simulink library "tpm"  (R2021b)
settings: Solver=VariableStepAuto  StartTime=0.0  StopTime=10.0  RelTol=1e-3
undefined symbols (not defined in the file or in its folder): ENUM_AN_LF, ENUM_AN_LR, ENUM_AN_RF, ENUM_AN_RR, ENUM_POWERSTA_OFF, ENUM_POWERSTA_OFFA, ENUM_POWERSTA_OFFC, ENUM_POWERSTA_ON, ENUM_POWERSTA_READY, ENUM_POWERSTA_STANDBY, ENUM_PWRSTASW_OFF, ENUM_PWRSTASW_OFFA, ENUM_PWRSTASW_OFFCHVCHRG, ENUM_PWRSTASW_STANDBY, KTPM_Delay_raw8, KTPM_WhlRotDir_enum_ovrdflg, KTPM_WhlRotDir_enum_ovrdval, TRUE, ZERO_FLOAT, ZERO_INT
libraries: simulink x58, hcu_lib x25, $bdroot x18
(part 5 of 8)

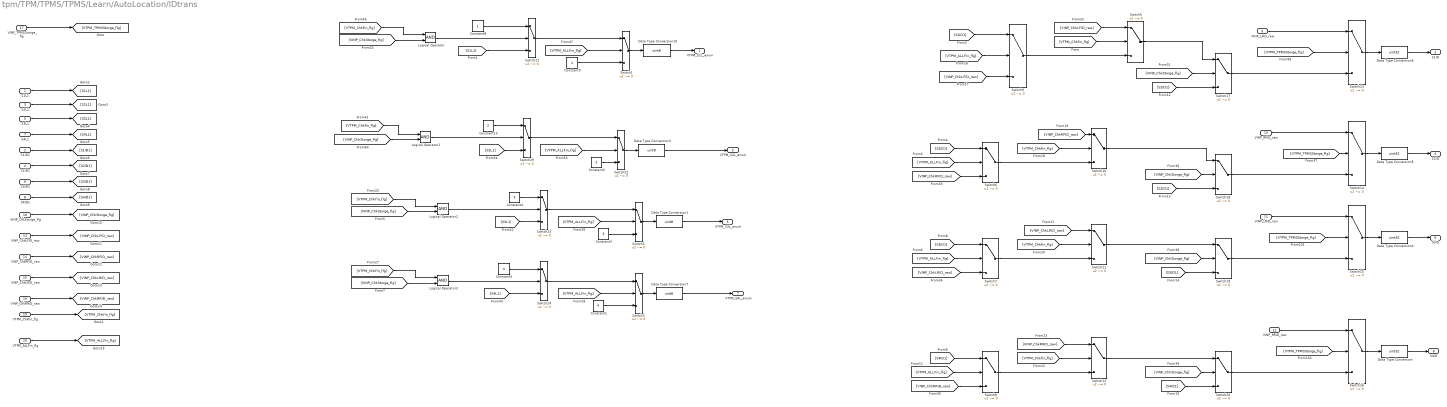
== system tpm/TPM/TPMS/TPMS/Learn/AutoLocation/IDtrans ==
  S1L1 : Inport
  S1ID1 : Inport  Port=2
  S2L1 : Inport  Port=3
  S2ID1 : Inport  Port=4
  S3L1 : Inport  Port=5
  S3ID1 : Inport  Port=6
  S4L1 : Inport  Port=7
  S4ID1 : Inport  Port=8
  VINP_LFID_raw : Inport  Port=9
  VINP_RFID_raw : Inport  Port=10
  VINP_LRID_raw : Inport  Port=11
  VINP_RRID_raw : Inport  Port=12
  VINP_ChkLFID_raw : Inport  Port=13
  VINP_ChkRFID_raw : Inport  Port=14
  VINP_ChkLRID_raw : Inport  Port=15
  VINP_ChkRRID_raw : Inport  Port=16
  VINP_TPMSStorge_flg : Inport  Port=17
  VINP_ChkStorge_flg : Inport  Port=18
  VTPM_Chkfin_flg : Inport  Port=19
  VTPM_ALLFin_flg : Inport  Port=20
  Constant1 : Constant  Value=4
  Constant13 : Constant  Value=2
  Constant2 : Constant  Value=2
  Constant3 : Constant  Value=3
  Constant4 : Constant  Value=3
  Constant5 : Constant  Value=4
  Constant8 : Constant
  Constant9 : Constant
  Data Type Conversion{,4..6} (4 alike) : DataTypeConversion  OutDataTypeStr=uint32
  Data Type Conversion{1,3,7,10} (4 alike) : DataTypeConversion  OutDataTypeStr=uint8
  Logical Operator{,1..3} (4 alike) : Logic  AllPortsSameDT=off  OutDataTypeStr=boolean
  Switch{1..3,5..24,29} (24 alike) : Switch  Criteria=u2 ~= 0
  VTPM_S1L_enum : Outport
  S1ID : Outport  Port=2
  VTPM_S2L_enum : Outport  Port=3
  S2ID : Outport  Port=4
  VTPM_S3L_enum : Outport  Port=5
  S3ID : Outport  Port=6
  VTPM_S4L_enum : Outport  Port=7
  S4ID : Outport  Port=8
  wires:
  Data Type Conversion4/1 -> S3ID/1
  Data Type Conversion6/1 -> S1ID/1
  Data Type Conversion/1 -> S4ID/1
  [VTPM_TPMSStorge_flg] -> Switch13/2
  Data Type Conversion5/1 -> S2ID/1
  VINP_TPMSStorge_flg/1 -> [VTPM_TPMSStorge_flg]
  S1L1/1 -> [S1L1]
  S2L1/1 -> [S2L1]
  S3L1/1 -> [S3L1]
  S4L1/1 -> [S4L1]
  S1ID1/1 -> [S1ID1]
  S2ID1/1 -> [S2ID1]
  S3ID1/1 -> [S3ID1]
  S4ID1/1 -> [S4ID1]
  VINP_LFID_raw/1 -> Switch13/1
  [VTPM_TPMSStorge_flg] -> Switch14/2
  Switch14/1 -> Data Type Conversion5/1
  Switch18/1 -> Switch14/3
  [VTPM_TPMSStorge_flg] -> Switch15/2
  VINP_LRID_raw/1 -> Switch15/1
  Switch19/1 -> Switch15/3
  Switch15/1 -> Data Type Conversion4/1
  VINP_RRID_raw/1 -> Switch16/1
  [VTPM_TPMSStorge_flg] -> Switch16/2
  Switch16/1 -> Data Type Conversion/1
  Switch13/1 -> Data Type Conversion6/1
  VINP_ChkStorge_flg/1 -> [VINP_ChkStorge_flg]
  VINP_ChkLFID_raw/1 -> [VINP_ChkLFID_raw]
  VINP_ChkRFID_raw/1 -> [VINP_ChkRFID_raw]
  VINP_ChkLRID_raw/1 -> [VINP_ChkLRID_raw]
  VINP_ChkRRID_raw/1 -> [VINP_ChkRRID_raw]
  [S1ID1] -> Switch17/3
  [VINP_ChkStorge_flg] -> Switch17/2
  [S2ID1] -> Switch18/3
  [VINP_ChkStorge_flg] -> Switch18/2
  [VINP_ChkStorge_flg] -> Switch19/2
  [S3ID1] -> Switch19/3
  [VINP_ChkStorge_flg] -> Switch20/2
  [S4ID1] -> Switch20/3
  Switch17/1 -> Switch13/3
  VINP_RFID_raw/1 -> Switch14/1
  Switch20/1 -> Switch16/3
  VTPM_ALLFin_flg/1 -> [VTPM_ALLFin_flg]
  VTPM_Chkfin_flg/1 -> [VTPM_Chkfin_flg]
  Switch5/1 -> Switch17/1
  [VTPM_Chkfin_flg] -> Switch5/2
  [VINP_ChkRFID_raw] -> Switch6/3
  [VTPM_ALLFin_flg] -> Switch6/2
  [S2ID1] -> Switch6/1
  [VINP_ChkLRID_raw] -> Switch7/3
  [VTPM_ALLFin_flg] -> Switch7/2
  [S3ID1] -> Switch7/1
  [S4ID1] -> Switch8/1
  [VINP_ChkRRID_raw] -> Switch8/3
  [VTPM_ALLFin_flg] -> Switch8/2
  [VTPM_ALLFin_flg] -> Switch9/2
  [S1ID1] -> Switch9/1
  [VINP_ChkLFID_raw] -> Switch9/3
  [VINP_ChkLFID_raw] -> Switch5/1
  Switch9/1 -> Switch5/3
  Switch10/1 -> Switch18/1
  [VTPM_Chkfin_flg] -> Switch10/2
  Switch6/1 -> Switch10/3
  [VINP_ChkRFID_raw] -> Switch10/1
  Switch11/1 -> Switch19/1
  Switch7/1 -> Switch11/3
  [VTPM_Chkfin_flg] -> Switch11/2
  [VINP_ChkLRID_raw] -> Switch11/1
  [VTPM_Chkfin_flg] -> Switch12/2
  Switch12/1 -> Switch20/1
  Switch8/1 -> Switch12/3
  [VINP_ChkRRID_raw] -> Switch12/1
  Switch1/1 -> Data Type Conversion10/1
  Data Type Conversion10/1 -> VTPM_S1L_enum/1
  [VTPM_ALLFin_flg] -> Switch1/2
  Switch21/1 -> Switch1/1
  Constant9/1 -> Switch1/3
  Constant8/1 -> Switch21/1
  Logical Operator/1 -> Switch21/2
  [VTPM_Chkfin_flg] -> Logical Operator/1
  [VINP_ChkStorge_flg] -> Logical Operator/2
  [S1L1] -> Switch21/3
  [VTPM_Chkfin_flg] -> Logical Operator1/1
  Switch29/1 -> Switch22/1
  Switch22/1 -> Data Type Conversion3/1
  Logical Operator1/1 -> Switch29/2
  [VTPM_ALLFin_flg] -> Switch22/2
  [VINP_ChkStorge_flg] -> Logical Operator1/2
  Data Type Conversion3/1 -> VTPM_S2L_enum/1
  Constant2/1 -> Switch22/3
  Constant13/1 -> Switch29/1
  [S2L1] -> Switch29/3
  [VTPM_Chkfin_flg] -> Logical Operator2/1
  Switch23/1 -> Switch2/1
  Switch2/1 -> Data Type Conversion1/1
  Logical Operator2/1 -> Switch23/2
  [VTPM_ALLFin_flg] -> Switch2/2
  [VINP_ChkStorge_flg] -> Logical Operator2/2
  Constant3/1 -> Switch2/3
  Data Type Conversion1/1 -> VTPM_S3L_enum/1
  Constant4/1 -> Switch23/1
  [S3L1] -> Switch23/3
  [VTPM_Chkfin_flg] -> Logical Operator3/1
  Switch24/1 -> Switch3/1
  Switch3/1 -> Data Type Conversion7/1
  Logical Operator3/1 -> Switch24/2
  [VTPM_ALLFin_flg] -> Switch3/2
  [VINP_ChkStorge_flg] -> Logical Operator3/2
  Data Type Conversion7/1 -> VTPM_S4L_enum/1
  Constant1/1 -> Switch3/3
  [S4L1] -> Switch24/3
  Constant5/1 -> Switch24/1

== system tpm/TPM/TPMS/TPMS/Learn/AutoLocation/Subsystem ==
  S1ID : Inport
  S2ID : Inport  Port=2
  S3ID : Inport  Port=3
  S4ID : Inport  Port=4
  VINP_TPMSResButt_flg : Inport  Port=5
  Enable : EnablePort
  Chart : Stateflow chart  TreatAsAtomicUnit=on
  VTPM_FlashS1ID_raw : Outport
  VTPM_FlashS2ID_raw : Outport  Port=2
  VTPM_FlashS3ID_raw : Outport  Port=3
  VTPM_FlashS4ID_raw : Outport  Port=4
  VTPM_FlashIDvalid_enum : Outport  Port=5
  wires:
  S4ID/1 -> Chart/4(S4ID)
  VINP_TPMSResButt_flg/1 -> Chart/5(VINP_TPMSResButt_flg)
  S3ID/1 -> Chart/3(S3ID)
  S2ID/1 -> Chart/2(S2ID)
  S1ID/1 -> Chart/1(S1ID)
  Chart/5(VTPM_FlashIDvalid_enum) -> VTPM_FlashIDvalid_enum/1
  Chart/4(VTPM_FlashS4ID_raw) -> VTPM_FlashS4ID_raw/1
  Chart/3(VTPM_FlashS3ID_raw) -> VTPM_FlashS3ID_raw/1
  Chart/2(VTPM_FlashS2ID_raw) -> VTPM_FlashS2ID_raw/1
  Chart/1(VTPM_FlashS1ID_raw) -> VTPM_FlashS1ID_raw/1

== system tpm/TPM/TPMS/TPMS/Learn/AutoLocation/WheelPosition ==
  VPMM_PowerSta_enum : Inport
  VINP_LFPulseCountV_flg : Inport  Port=2
  VTPM_LFWhlRotDir_enum : Inport  Port=3
  VINP_LFPulseCount_cnt : Inport  Port=4
  VINP_RFPulseCountV_flg : Inport  Port=5
  VTPM_RFWhlRotDir_enum : Inport  Port=6
  VINP_RFPulseCount_cnt : Inport  Port=7
  VINP_LRPulseCountV_flg : Inport  Port=8
  VTPM_LRWhlRotDir_enum : Inport  Port=9
  VINP_LRPulseCount_cnt : Inport  Port=10
  VINP_RRPulseCountV_flg : Inport  Port=11
  VTPM_RRWhlRotDir_enum : Inport  Port=12
  VINP_RRPulseCount_cnt : Inport  Port=13
  Chart1 : Stateflow chart
      settings: PortSchema="{\"entries\":[{\"content\":{\"sides\":[{\"content\":{\"connectorIds\":[\"In1\",\"In3\",\"In4\",\"In2\"]},\"type\":\"ConnectorPlacement.EquallySpacedRectSide\",\"uuid\":\"75b213f6-e1d2-4b51-b3b2-bb9425a07129\"},{\"content\":{\"connectorIds\":[\"Out1\"],\"side\":\"RIGHT\"},\"type\":\"ConnectorPlacement.EquallySpacedRectSide\",\"uuid\":\"38a0f576-9623-4928-9f9d-a0457630f06b\"},{\"content\":{\"connectorIds\":[],\"side\":\"TOP\"},\"type\":\"ConnectorPlacement.EquallySpacedRectSide\",\"uuid\":\"5f96c838-eaaa-41a3-a60b-23098d5837b3\"}]},\"type\":\"ConnectorPlacement.EquallySpacedConnector\",\"uuid\":\"5c398a97-3ae6-4872-b8e8-e03a196625be\"}],\"packageUris\":[\"http://schema.mathworks.com/mf0/Connector/R2020b\"],\"version\":\"1.0\"}"
  Chart2 : Stateflow chart
      settings: PortSchema="{\"entries\":[{\"content\":{\"sides\":[{\"content\":{\"connectorIds\":[\"In1\",\"In3\",\"In4\",\"In2\"]},\"type\":\"ConnectorPlacement.EquallySpacedRectSide\",\"uuid\":\"75b213f6-e1d2-4b51-b3b2-bb9425a07129\"},{\"content\":{\"connectorIds\":[\"Out1\"],\"side\":\"RIGHT\"},\"type\":\"ConnectorPlacement.EquallySpacedRectSide\",\"uuid\":\"38a0f576-9623-4928-9f9d-a0457630f06b\"},{\"content\":{\"connectorIds\":[],\"side\":\"TOP\"},\"type\":\"ConnectorPlacement.EquallySpacedRectSide\",\"uuid\":\"5f96c838-eaaa-41a3-a60b-23098d5837b3\"}]},\"type\":\"ConnectorPlacement.EquallySpacedConnector\",\"uuid\":\"5c398a97-3ae6-4872-b8e8-e03a196625be\"}],\"packageUris\":[\"http://schema.mathworks.com/mf0/Connector/R2020b\"],\"version\":\"1.0\"}"
  Chart3 : Stateflow chart
      settings: PortSchema="{\"entries\":[{\"content\":{\"sides\":[{\"content\":{\"connectorIds\":[\"In1\",\"In3\",\"In4\",\"In2\"]},\"type\":\"ConnectorPlacement.EquallySpacedRectSide\",\"uuid\":\"75b213f6-e1d2-4b51-b3b2-bb9425a07129\"},{\"content\":{\"connectorIds\":[\"Out1\"],\"side\":\"RIGHT\"},\"type\":\"ConnectorPlacement.EquallySpacedRectSide\",\"uuid\":\"38a0f576-9623-4928-9f9d-a0457630f06b\"},{\"content\":{\"connectorIds\":[],\"side\":\"TOP\"},\"type\":\"ConnectorPlacement.EquallySpacedRectSide\",\"uuid\":\"5f96c838-eaaa-41a3-a60b-23098d5837b3\"}]},\"type\":\"ConnectorPlacement.EquallySpacedConnector\",\"uuid\":\"5c398a97-3ae6-4872-b8e8-e03a196625be\"}],\"packageUris\":[\"http://schema.mathworks.com/mf0/Connector/R2020b\"],\"version\":\"1.0\"}"
  Chart5 : Stateflow chart
      settings: PortSchema="{\"entries\":[{\"content\":{\"sides\":[{\"content\":{\"connectorIds\":[\"In1\",\"In3\",\"In4\",\"In2\"]},\"type\":\"ConnectorPlacement.EquallySpacedRectSide\",\"uuid\":\"75b213f6-e1d2-4b51-b3b2-bb9425a07129\"},{\"content\":{\"connectorIds\":[\"Out1\"],\"side\":\"RIGHT\"},\"type\":\"ConnectorPlacement.EquallySpacedRectSide\",\"uuid\":\"38a0f576-9623-4928-9f9d-a0457630f06b\"},{\"content\":{\"connectorIds\":[],\"side\":\"TOP\"},\"type\":\"ConnectorPlacement.EquallySpacedRectSide\",\"uuid\":\"5f96c838-eaaa-41a3-a60b-23098d5837b3\"}]},\"type\":\"ConnectorPlacement.EquallySpacedConnector\",\"uuid\":\"5c398a97-3ae6-4872-b8e8-e03a196625be\"}],\"packageUris\":[\"http://schema.mathworks.com/mf0/Connector/R2020b\"],\"version\":\"1.0\"}"
  Subsystem : Subsystem
  Subsystem1 : Subsystem
  Subsystem2 : Subsystem
  Subsystem3 : Subsystem
  VTPM_RFWP_raw16 : Outport
  VTPM_LRWP_raw16 : Outport  Port=2
  VTPM_RRWP_raw16 : Outport  Port=3
  VTPM_LFWP_raw16 : Outport  Port=4
  wires:
  VPMM_PowerSta_enum/1 -> [VPMM_PowerSta_enum]
  [VPMM_PowerSta_enum] -> Chart1/1(VPMM_PowerSta_enum)
  [VPMM_PowerSta_enum] -> Chart2/1(VPMM_PowerSta_enum)
  [VPMM_PowerSta_enum] -> Chart3/1(VPMM_PowerSta_enum)
  VINP_LFPulseCountV_flg/1 -> Chart1/3(VINP_LFPulseCountV_flg)
  VTPM_LFWhlRotDir_enum/1 -> Chart1/4(VTPM_LFWhlRotDir_enum)
  VINP_LFPulseCount_cnt/1 -> Chart1/2(VINP_LFPulseCount_cnt)
  VINP_RFPulseCountV_flg/1 -> Chart2/3(VINP_RFPulseCountV_flg)
  VTPM_RFWhlRotDir_enum/1 -> Chart2/4(VTPM_RFWhlRotDir_enum)
  VINP_RFPulseCount_cnt/1 -> Chart2/2(VINP_RFPulseCount_cnt)
  VINP_LRPulseCountV_flg/1 -> Chart3/3(VINP_LRPulseCountV_flg)
  VTPM_LRWhlRotDir_enum/1 -> Chart3/4(VTPM_LRWhlRotDir_enum)
  VINP_LRPulseCount_cnt/1 -> Chart3/2(VINP_LRPulseCount_cnt)
  Subsystem/1(VTPM_LFWP_raw16) -> VTPM_LFWP_raw16/1
  Subsystem1/1(VTPM_RFWP_raw16) -> VTPM_RFWP_raw16/1
  Subsystem2/1(VTPM_LRWP_raw16) -> VTPM_LRWP_raw16/1
  Subsystem3/1(VTPM_RRWP_raw16) -> VTPM_RRWP_raw16/1
  Chart1/1(VTPM_LFWpos_raw) -> Subsystem/1(VTPM_LFWpos_raw)  "VTPM_LFWpos_raw"
  Chart2/1(VTPM_RFWpos_raw) -> Subsystem1/1(VTPM_RFWpos_raw)  "VTPM_RFWpos_raw"
  Chart3/1(VTPM_LRWpos_raw) -> Subsystem2/1(VTPM_LRWpos_raw)  "VTPM_LRWpos_raw"
  [VPMM_PowerSta_enum] -> Chart5/1(VPMM_PowerSta_enum)
  VINP_RRPulseCountV_flg/1 -> Chart5/3(VINP_RRPulseCountV_flg)
  VTPM_RRWhlRotDir_enum/1 -> Chart5/4(VTPM_RRWhlRotDir_enum)
  VINP_RRPulseCount_cnt/1 -> Chart5/2(VINP_RRPulseCount_cnt)
  Chart5/1(VTPM_RRWpos_raw) -> Subsystem3/1(VTPM_RRWpos_raw)  "VTPM_RRWpos_raw"

== system tpm/TPM/TPMS/TPMS/Send/Alarm/LFTHighWarn ==
  VTPM_LFWheelTemp_C : Inport
  Compare To Constant : simulink/Logic and Bit Operations/Compare To Constant  relop=>=  const=90  OutDataTypeStr=boolean
  Compare To Constant1 : simulink/Logic and Bit Operations/Compare To Constant  relop=>=  const=84  OutDataTypeStr=boolean
  Logical Operator1 : Logic  Operator=OR  AllPortsSameDT=off  OutDataTypeStr=boolean
  Logical Operator2 : Logic  AllPortsSameDT=off  OutDataTypeStr=boolean
  Unit Delay : UnitDelay  SampleTime=-1  HasFrameUpgradeWarning=on
  VTPM_LFWheelTmpIndi_flg : Outport
  wires:
  Compare To Constant/1 -> Logical Operator1/1
  Unit Delay/1 -> Logical Operator2/2
  Logical Operator2/1 -> Logical Operator1/2
  Logical Operator1/1 -> VTPM_LFWheelTmpIndi_flg/1, Unit Delay/1
  Compare To Constant1/1 -> Logical Operator2/1
  VTPM_LFWheelTemp_C/1 -> Compare To Constant/1, Compare To Constant1/1

== system tpm/TPM/TPMS/TPMS/Send/Alarm/LRTHighWarn ==
  VTPM_LRWheelTemp_C : Inport
  Compare To Constant : simulink/Logic and Bit Operations/Compare To Constant  relop=>=  const=90  OutDataTypeStr=boolean
  Compare To Constant1 : simulink/Logic and Bit Operations/Compare To Constant  relop=>=  const=84  OutDataTypeStr=boolean
  Logical Operator1 : Logic  Operator=OR  AllPortsSameDT=off  OutDataTypeStr=boolean
  Logical Operator2 : Logic  AllPortsSameDT=off  OutDataTypeStr=boolean
  Unit Delay : UnitDelay  SampleTime=-1  HasFrameUpgradeWarning=on
  VTPM_LRWheelTmpIndi_flg : Outport
  wires:
  Compare To Constant/1 -> Logical Operator1/1
  Unit Delay/1 -> Logical Operator2/2
  Logical Operator2/1 -> Logical Operator1/2
  Logical Operator1/1 -> VTPM_LRWheelTmpIndi_flg/1, Unit Delay/1
  Compare To Constant1/1 -> Logical Operator2/1
  VTPM_LRWheelTemp_C/1 -> Compare To Constant/1, Compare To Constant1/1

== system tpm/TPM/TPMS/TPMS/Send/Alarm/RFTHighWarn ==
  VTPM_RFWheelTemp_C : Inport
  Compare To Constant : simulink/Logic and Bit Operations/Compare To Constant  relop=>=  const=90  OutDataTypeStr=boolean
  Compare To Constant1 : simulink/Logic and Bit Operations/Compare To Constant  relop=>=  const=84  OutDataTypeStr=boolean
  Logical Operator1 : Logic  Operator=OR  AllPortsSameDT=off  OutDataTypeStr=boolean
  Logical Operator2 : Logic  AllPortsSameDT=off  OutDataTypeStr=boolean
  Unit Delay : UnitDelay  SampleTime=-1  HasFrameUpgradeWarning=on
  VTPM_RFWheelTmpIndi_flg : Outport
  wires:
  VTPM_RFWheelTemp_C/1 -> Compare To Constant1/1, Compare To Constant/1
  Compare To Constant1/1 -> Logical Operator2/1
  Logical Operator1/1 -> VTPM_RFWheelTmpIndi_flg/1, Unit Delay/1
  Logical Operator2/1 -> Logical Operator1/2
  Unit Delay/1 -> Logical Operator2/2
  Compare To Constant/1 -> Logical Operator1/1

== system tpm/TPM/TPMS/TPMS/Send/Alarm/RRTHighWarn ==
  VTPM_RRWheelTemp_C : Inport
  Compare To Constant : simulink/Logic and Bit Operations/Compare To Constant  relop=>=  const=90  OutDataTypeStr=boolean
  Compare To Constant1 : simulink/Logic and Bit Operations/Compare To Constant  relop=>=  const=84  OutDataTypeStr=boolean
  Logical Operator1 : Logic  Operator=OR  AllPortsSameDT=off  OutDataTypeStr=boolean
  Logical Operator2 : Logic  AllPortsSameDT=off  OutDataTypeStr=boolean
  Unit Delay : UnitDelay  SampleTime=-1  HasFrameUpgradeWarning=on
  VTPM_RRWheelTmpIndi_flg : Outport
  wires:
  VTPM_RRWheelTemp_C/1 -> Compare To Constant1/1, Compare To Constant/1
  Compare To Constant1/1 -> Logical Operator2/1
  Logical Operator1/1 -> VTPM_RRWheelTmpIndi_flg/1, Unit Delay/1
  Logical Operator2/1 -> Logical Operator1/2
  Unit Delay/1 -> Logical Operator2/2
  Compare To Constant/1 -> Logical Operator1/1

== system tpm/TPM/TPMS/TPMS/Send/DATA/LocationSW ==
  VTPM_S1ID_raw32 : Inport
  VTPM_S2ID_raw32 : Inport  Port=2
  VTPM_S3ID_raw32 : Inport  Port=3
  VTPM_S4ID_raw32 : Inport  Port=4
  VINP_IDin_raw32 : Inport  Port=5
  VTPM_S1L_enum : Inport  Port=6
  VTPM_S2L_enum : Inport  Port=7
  VTPM_S3L_enum : Inport  Port=8
  VTPM_S4L_enum : Inport  Port=9
  VINP_DATAin_flg : Inport  Port=10
  VTPM_IDLOCK_flg : Inport  Port=11
  Chart1 : Stateflow chart  TreatAsAtomicUnit=on
  VTPM_LFSW_flg : Outport
  VTPM_RFSW_flg : Outport  Port=2
  VTPM_LRSW_flg : Outport  Port=3
  VTPM_RRSW_flg : Outport  Port=4
  wires:
  VTPM_S1ID_raw32/1 -> Chart1/1(VTPM_S1ID_raw32)
  VTPM_S1L_enum/1 -> Chart1/2(VTPM_S1L_enum)
  VTPM_S2ID_raw32/1 -> Chart1/3(VTPM_S2ID_raw32)
  VTPM_S2L_enum/1 -> Chart1/4(VTPM_S2L_enum)
  VTPM_S3ID_raw32/1 -> Chart1/5(VTPM_S3ID_raw32)
  VTPM_S3L_enum/1 -> Chart1/6(VTPM_S3L_enum)
  VTPM_S4ID_raw32/1 -> Chart1/7(VTPM_S4ID_raw32)
  VTPM_S4L_enum/1 -> Chart1/8(VTPM_S4L_enum)
  VINP_IDin_raw32/1 -> Chart1/9(VINP_IDin_raw32)
  VINP_DATAin_flg/1 -> Chart1/10(VINP_DATAin_flg)
  Chart1/1(VTPM_LFSW_flg) -> VTPM_LFSW_flg/1
  Chart1/2(VTPM_RFSW_flg) -> VTPM_RFSW_flg/1
  Chart1/3(VTPM_LRSW_flg) -> VTPM_LRSW_flg/1
  Chart1/4(VTPM_RRSW_flg) -> VTPM_RRSW_flg/1
  VTPM_IDLOCK_flg/1 -> Chart1/11(VTPM_IDLOCK_flg)

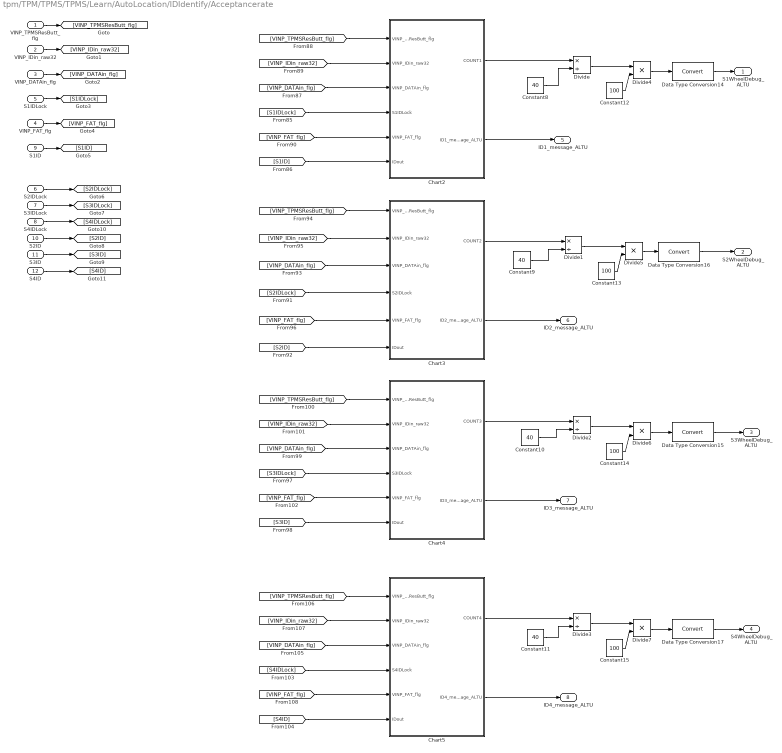
== system tpm/TPM/TPMS/TPMS/Learn/AutoLocation/IDIdentify/Acceptancerate ==
  VINP_TPMSResButt_flg : Inport
  VINP_IDin_raw32 : Inport  Port=2
  VINP_DATAin_flg : Inport  Port=3
  VINP_FAT_flg : Inport  Port=4
  S1IDLock : Inport  Port=5
  S2IDLock : Inport  Port=6
  S3IDLock : Inport  Port=7
  S4IDLock : Inport  Port=8
  S1ID : Inport  Port=9
  S2ID : Inport  Port=10
  S3ID : Inport  Port=11
  S4ID : Inport  Port=12
  Chart2 : Stateflow chart  TreatAsAtomicUnit=on
      settings: PortSchema="{\"entries\":[{\"content\":{\"sides\":[{\"content\":{\"connectorIds\":[\"In2\",\"In1\",\"In3\",\"In4\",\"In5\",\"In6\"]},\"type\":\"ConnectorPlacement.EquallySpacedRectSide\",\"uuid\":\"0106c0c7-b0dd-4985-8477-027279f2cfbe\"},{\"content\":{\"connectorIds\":[\"Out1\",\"Out2\"],\"side\":\"RIGHT\"},\"type\":\"ConnectorPlacement.EquallySpacedRectSide\",\"uuid\":\"38b36b5e-8790-43f5-89a8-de723ff40088\"},{\"content\":{\"connectorIds\":[],\"side\":\"TOP\"},\"type\":\"ConnectorPlacement.EquallySpacedRectSide\",\"uuid\":\"aa12a430-979d-4bba-b5af-88414204d80d\"}]},\"type\":\"ConnectorPlacement.EquallySpacedConnector\",\"uuid\":\"9f6249c4-6459-404e-8830-3ea500254943\"}],\"packageUris\":[\"http://schema.mathworks.com/mf0/Connector/R2020b\"],\"version\":\"1.0\"}"
  Chart3 : Stateflow chart  TreatAsAtomicUnit=on
      settings: PortSchema="{\"entries\":[{\"content\":{\"sides\":[{\"content\":{\"connectorIds\":[\"In2\",\"In1\",\"In3\",\"In6\",\"In4\",\"In5\"]},\"type\":\"ConnectorPlacement.EquallySpacedRectSide\",\"uuid\":\"0106c0c7-b0dd-4985-8477-027279f2cfbe\"},{\"content\":{\"connectorIds\":[\"Out2\",\"Out1\"],\"side\":\"RIGHT\"},\"type\":\"ConnectorPlacement.EquallySpacedRectSide\",\"uuid\":\"38b36b5e-8790-43f5-89a8-de723ff40088\"},{\"content\":{\"connectorIds\":[],\"side\":\"TOP\"},\"type\":\"ConnectorPlacement.EquallySpacedRectSide\",\"uuid\":\"aa12a430-979d-4bba-b5af-88414204d80d\"}]},\"type\":\"ConnectorPlacement.EquallySpacedConnector\",\"uuid\":\"9f6249c4-6459-404e-8830-3ea500254943\"}],\"packageUris\":[\"http://schema.mathworks.com/mf0/Connector/R2020b\"],\"version\":\"1.0\"}"
  Chart4 : Stateflow chart  TreatAsAtomicUnit=on
      settings: PortSchema="{\"entries\":[{\"content\":{\"sides\":[{\"content\":{\"connectorIds\":[\"In2\",\"In1\",\"In3\",\"In4\",\"In5\",\"In6\"]},\"type\":\"ConnectorPlacement.EquallySpacedRectSide\",\"uuid\":\"0106c0c7-b0dd-4985-8477-027279f2cfbe\"},{\"content\":{\"connectorIds\":[\"Out1\",\"Out2\"],\"side\":\"RIGHT\"},\"type\":\"ConnectorPlacement.EquallySpacedRectSide\",\"uuid\":\"38b36b5e-8790-43f5-89a8-de723ff40088\"},{\"content\":{\"connectorIds\":[],\"side\":\"TOP\"},\"type\":\"ConnectorPlacement.EquallySpacedRectSide\",\"uuid\":\"aa12a430-979d-4bba-b5af-88414204d80d\"}]},\"type\":\"ConnectorPlacement.EquallySpacedConnector\",\"uuid\":\"9f6249c4-6459-404e-8830-3ea500254943\"}],\"packageUris\":[\"http://schema.mathworks.com/mf0/Connector/R2020b\"],\"version\":\"1.0\"}"
  Chart5 : Stateflow chart  TreatAsAtomicUnit=on
      settings: PortSchema="{\"entries\":[{\"content\":{\"sides\":[{\"content\":{\"connectorIds\":[\"In2\",\"In1\",\"In3\",\"In4\",\"In5\",\"In6\"]},\"type\":\"ConnectorPlacement.EquallySpacedRectSide\",\"uuid\":\"0106c0c7-b0dd-4985-8477-027279f2cfbe\"},{\"content\":{\"connectorIds\":[\"Out1\",\"Out2\"],\"side\":\"RIGHT\"},\"type\":\"ConnectorPlacement.EquallySpacedRectSide\",\"uuid\":\"38b36b5e-8790-43f5-89a8-de723ff40088\"},{\"content\":{\"connectorIds\":[],\"side\":\"TOP\"},\"type\":\"ConnectorPlacement.EquallySpacedRectSide\",\"uuid\":\"aa12a430-979d-4bba-b5af-88414204d80d\"}]},\"type\":\"ConnectorPlacement.EquallySpacedConnector\",\"uuid\":\"9f6249c4-6459-404e-8830-3ea500254943\"}],\"packageUris\":[\"http://schema.mathworks.com/mf0/Connector/R2020b\"],\"version\":\"1.0\"}"
  Constant{8..11} (4 alike) : Constant  Value=40
  Constant{12..15} (4 alike) : Constant  Value=100
  Data Type Conversion{14..17} (4 alike) : DataTypeConversion
  Divide{,1..3} (4 alike) : Product  Inputs=*/
  Divide{4..7} (4 alike) : Product  Inputs=**
  S1WheelDebug_ALTU : Outport
  S2WheelDebug_ALTU : Outport  Port=2
  S3WheelDebug_ALTU : Outport  Port=3
  S4WheelDebug_ALTU : Outport  Port=4
  ID1_message_ALTU : Outport  Port=5
  ID2_message_ALTU : Outport  Port=6
  ID3_message_ALTU : Outport  Port=7
  ID4_message_ALTU : Outport  Port=8
  wires:
  Chart3/2(COUNT2) -> Divide1/1
  [VINP_FAT_flg] -> Chart2/5(VINP_FAT_flg)
  [VINP_DATAin_flg] -> Chart3/3(VINP_DATAin_flg)
  Chart2/1(COUNT1) -> Divide/1
  Constant9/1 -> Divide1/2
  [VINP_IDin_raw32] -> Chart4/1(VINP_IDin_raw32)
  [VINP_TPMSResButt_flg] -> Chart2/2(VINP_TPMSResButt_flg)
  Constant12/1 -> Divide4/2
  Chart5/2(ID4_message_ALTU) -> ID4_message_ALTU/1
  Chart4/1(COUNT3) -> Divide2/1
  Constant8/1 -> Divide/2
  Constant15/1 -> Divide7/2
  Divide2/1 -> Divide6/1
  [VINP_DATAin_flg] -> Chart4/3(VINP_DATAin_flg)
  [VINP_IDin_raw32] -> Chart3/1(VINP_IDin_raw32)
  [VINP_TPMSResButt_flg] -> Chart3/2(VINP_TPMSResButt_flg)
  [VINP_FAT_flg] -> Chart5/5(VINP_FAT_flg)
  [VINP_IDin_raw32] -> Chart5/1(VINP_IDin_raw32)
  [S1ID] -> Chart2/6(IDout)
  Chart3/1(ID2_message_ALTU) -> ID2_message_ALTU/1
  [S2ID] -> Chart3/5(IDout)
  Chart4/2(ID3_message_ALTU) -> ID3_message_ALTU/1
  [S3IDLock] -> Chart4/4(S3IDLock)
  [VINP_TPMSResButt_flg] -> Chart4/2(VINP_TPMSResButt_flg)
  Divide1/1 -> Divide5/1
  [VINP_DATAin_flg] -> Chart5/3(VINP_DATAin_flg)
  Constant10/1 -> Divide2/2
  [VINP_TPMSResButt_flg] -> Chart5/2(VINP_TPMSResButt_flg)
  Divide3/1 -> Divide7/1
  [S2IDLock] -> Chart3/6(S2IDLock)
  [VINP_IDin_raw32] -> Chart2/1(VINP_IDin_raw32)
  Data Type Conversion16/1 -> S2WheelDebug_ALTU/1
  [VINP_FAT_flg] -> Chart3/4(VINP_FAT_flg)
  [S4IDLock] -> Chart5/4(S4IDLock)
  Constant13/1 -> Divide5/2
  [S1IDLock] -> Chart2/4(S1IDLock)
  Data Type Conversion15/1 -> S3WheelDebug_ALTU/1
  Data Type Conversion17/1 -> S4WheelDebug_ALTU/1
  Chart5/1(COUNT4) -> Divide3/1
  Divide5/1 -> Data Type Conversion16/1
  [S4ID] -> Chart5/6(IDout)
  [VINP_DATAin_flg] -> Chart2/3(VINP_DATAin_flg)
  Divide4/1 -> Data Type Conversion14/1
  [S3ID] -> Chart4/6(IDout)
  Constant11/1 -> Divide3/2
  Constant14/1 -> Divide6/2
  Divide6/1 -> Data Type Conversion15/1
  Chart2/2(ID1_message_ALTU) -> ID1_message_ALTU/1
  Divide/1 -> Divide4/1
  Divide7/1 -> Data Type Conversion17/1
  [VINP_FAT_flg] -> Chart4/5(VINP_FAT_flg)
  Data Type Conversion14/1 -> S1WheelDebug_ALTU/1
  VINP_TPMSResButt_flg/1 -> [VINP_TPMSResButt_flg]
  VINP_IDin_raw32/1 -> [VINP_IDin_raw32]
  VINP_DATAin_flg/1 -> [VINP_DATAin_flg]
  S1IDLock/1 -> [S1IDLock]
  VINP_FAT_flg/1 -> [VINP_FAT_flg]
  S1ID/1 -> [S1ID]
  S2IDLock/1 -> [S2IDLock]
  S3IDLock/1 -> [S3IDLock]
  S2ID/1 -> [S2ID]
  S3ID/1 -> [S3ID]
  S4ID/1 -> [S4ID]
  S4IDLock/1 -> [S4IDLock]

== system tpm/TPM/TPMS/TPMS/Learn/AutoLocation/IDIdentify/Enabled Subsystem ==
  VINP_TPMSResButt_flg : Inport
  VTPM_LFS1_cnt : Inport  Port=2
  VTPM_RFS1_cnt : Inport  Port=3
  VTPM_LRS1_cnt : Inport  Port=4
  VTPM_RRS1_cnt : Inport  Port=5
  VTPM_LFS2_cnt : Inport  Port=6
  VTPM_RFS2_cnt : Inport  Port=7
  VTPM_LRS2_cnt : Inport  Port=8
  VTPM_RRS2_cnt : Inport  Port=9
  VTPM_LFS3_cnt : Inport  Port=10
  VTPM_RFS3_cnt : Inport  Port=11
  VTPM_LRS3_cnt : Inport  Port=12
  VTPM_RRS3_cnt : Inport  Port=13
  VTPM_LFS4_cnt : Inport  Port=14
  VTPM_RFS4_cnt : Inport  Port=15
  VTPM_LRS4_cnt : Inport  Port=16
  VTPM_RRS4_cnt : Inport  Port=17
  Enable : EnablePort
  Data Type Conversion{,1..19} (20 alike) : DataTypeConversion  OutDataTypeStr=uint8
  MATLAB Function : MATLAB Function  TreatAsAtomicUnit=on
  S1L : Outport
  S2L : Outport  Port=2
  S3L : Outport  Port=3
  S4L : Outport  Port=4
  wires:
  VTPM_LFS1_cnt/1 -> Data Type Conversion4/1
  VTPM_RFS1_cnt/1 -> Data Type Conversion5/1
  VTPM_LRS1_cnt/1 -> Data Type Conversion6/1
  VTPM_RRS1_cnt/1 -> Data Type Conversion7/1
  VTPM_LFS2_cnt/1 -> Data Type Conversion8/1
  VTPM_RFS2_cnt/1 -> Data Type Conversion9/1
  VTPM_LRS2_cnt/1 -> Data Type Conversion10/1
  VTPM_RRS2_cnt/1 -> Data Type Conversion11/1
  VTPM_LFS3_cnt/1 -> Data Type Conversion12/1
  VTPM_RFS3_cnt/1 -> Data Type Conversion13/1
  VTPM_LRS3_cnt/1 -> Data Type Conversion14/1
  VTPM_RRS3_cnt/1 -> Data Type Conversion15/1
  VTPM_LFS4_cnt/1 -> Data Type Conversion16/1
  VTPM_RFS4_cnt/1 -> Data Type Conversion17/1
  VTPM_LRS4_cnt/1 -> Data Type Conversion18/1
  VTPM_RRS4_cnt/1 -> Data Type Conversion19/1
  Data Type Conversion/1 -> S1L/1
  Data Type Conversion1/1 -> S2L/1
  Data Type Conversion2/1 -> S3L/1
  Data Type Conversion3/1 -> S4L/1
  Data Type Conversion4/1 -> MATLAB Function/2(VTPM_LFS1_cnt)
  Data Type Conversion5/1 -> MATLAB Function/3(VTPM_RFS1_cnt)
  Data Type Conversion6/1 -> MATLAB Function/4(VTPM_LRS1_cnt)
  Data Type Conversion7/1 -> MATLAB Function/5(VTPM_RRS1_cnt)
  Data Type Conversion8/1 -> MATLAB Function/6(VTPM_LFS2_cnt)
  Data Type Conversion9/1 -> MATLAB Function/7(VTPM_RFS2_cnt)
  Data Type Conversion10/1 -> MATLAB Function/8(VTPM_LRS2_cnt)
  Data Type Conversion11/1 -> MATLAB Function/9(VTPM_RRS2_cnt)
  Data Type Conversion12/1 -> MATLAB Function/10(VTPM_LFS3_cnt)
  Data Type Conversion13/1 -> MATLAB Function/11(VTPM_RFS3_cnt)
  Data Type Conversion14/1 -> MATLAB Function/12(VTPM_LRS3_cnt)
  Data Type Conversion15/1 -> MATLAB Function/13(VTPM_RRS3_cnt)
  Data Type Conversion16/1 -> MATLAB Function/14(VTPM_LFS4_cnt)
  Data Type Conversion17/1 -> MATLAB Function/15(VTPM_RFS4_cnt)
  Data Type Conversion18/1 -> MATLAB Function/16(VTPM_LRS4_cnt)
  Data Type Conversion19/1 -> MATLAB Function/17(VTPM_RRS4_cnt)
  VINP_TPMSResButt_flg/1 -> MATLAB Function/1(VINP_TPMSResButt_flg)
  MATLAB Function/1(S1L) -> Data Type Conversion/1
  MATLAB Function/4(S4L) -> Data Type Conversion3/1
  MATLAB Function/3(S3L) -> Data Type Conversion2/1
  MATLAB Function/2(S2L) -> Data Type Conversion1/1

== system tpm/TPM/TPMS/TPMS/Learn/AutoLocation/IDIdentify/Subsystem1 ==
  VINP_DATAin_flg : Inport
  VINP_TPMSResButt_flg : Inport  Port=2
  VINP_IDin_raw32 : Inport  Port=3
  VTPM_LFWP_raw16 : Inport  Port=4
  VTPM_RFWP_raw16 : Inport  Port=5
  VTPM_LRWP_raw16 : Inport  Port=6
  VTPM_RRWP_raw16 : Inport  Port=7
  VPMM_PowerSta_enum : Inport  Port=8
  VINP_VehSpeed_kph : Inport  Port=9
  VINP_S2ID_raw : Inport  Port=10
  Add : Sum
  Chart : Stateflow chart  TreatAsAtomicUnit=on
      settings: PortSchema="{\"entries\":[{\"content\":{\"sides\":[{\"content\":{\"connectorIds\":[\"In1\",\"In2\",\"In3\",\"In5\",\"In7\",\"In4\",\"In6\"]},\"type\":\"ConnectorPlacement.EquallySpacedRectSide\",\"uuid\":\"84bbdee3-6a13-4113-bc08-a0b87ba22909\"},{\"content\":{\"connectorIds\":[\"Out5\",\"Out1\",\"Out4\",\"Out2\",\"Out3\"],\"side\":\"RIGHT\"},\"type\":\"ConnectorPlacement.EquallySpacedRectSide\",\"uuid\":\"b8796851-ab69-429f-9540-9571864c98e0\"},{\"content\":{\"connectorIds\":[],\"side\":\"TOP\"},\"type\":\"ConnectorPlacement.EquallySpacedRectSide\",\"uuid\":\"52bdbec4-409e-4a9a-a4bb-373a9525aed8\"}]},\"type\":\"ConnectorPlacement.EquallySpacedConnector\",\"uuid\":\"6e0a7370-38f8-4d4e-a3e7-eb2ef4c24b0f\"}],\"packageUris\":[\"http://schema.mathworks.com/mf0/Connector/R2020b\"],\"version\":\"1.0\"}"
  Chart1 : Stateflow chart  TreatAsAtomicUnit=on
      settings: PortSchema="{\"entries\":[{\"content\":{\"sides\":[{\"content\":{\"connectorIds\":[\"In2\",\"In1\",\"In3\",\"In4\",\"In5\",\"In6\"]},\"type\":\"ConnectorPlacement.EquallySpacedRectSide\",\"uuid\":\"0106c0c7-b0dd-4985-8477-027279f2cfbe\"},{\"content\":{\"connectorIds\":[\"Out1\",\"Out2\",\"Out3\",\"Out4\",\"Out5\"],\"side\":\"RIGHT\"},\"type\":\"ConnectorPlacement.EquallySpacedRectSide\",\"uuid\":\"38b36b5e-8790-43f5-89a8-de723ff40088\"},{\"content\":{\"connectorIds\":[],\"side\":\"TOP\"},\"type\":\"ConnectorPlacement.EquallySpacedRectSide\",\"uuid\":\"aa12a430-979d-4bba-b5af-88414204d80d\"}]},\"type\":\"ConnectorPlacement.EquallySpacedConnector\",\"uuid\":\"9f6249c4-6459-404e-8830-3ea500254943\"}],\"packageUris\":[\"http://schema.mathworks.com/mf0/Connector/R2020b\"],\"version\":\"1.0\"}"
  Constant : Constant  Value=ZERO_INT
  Constant18 : Constant  Value=0
  Data Type Conversion10 : DataTypeConversion  OutDataTypeStr=uint32
  Detect Increase : simulink/Logic and Bit Operations/Detect Increase  vinit=0.0  OutDataTypeStr=boolean
  Enabled Subsystem1 : Subsystem  TreatAsAtomicUnit=on
  Enabled Subsystem2 : Subsystem  TreatAsAtomicUnit=on
  Enabled Subsystem3 : Subsystem  TreatAsAtomicUnit=on
  Enabled Subsystem5 : Subsystem  TreatAsAtomicUnit=on
  Logical Operator : Logic  Operator=OR  AllPortsSameDT=off  OutDataTypeStr=boolean
  NOT : Logic  Operator=NOT  IconShape=distinctive  AllPortsSameDT=off  OutDataTypeStr=boolean
  Relational Operator : RelationalOperator  Operator=~=  OutDataTypeStr=boolean  RndMeth=Simplest
  Switch5 : Switch  Criteria=u2 > Threshold
  Unit Delay1 : UnitDelay  SampleTime=-1  HasFrameUpgradeWarning=on
  IDOut : Outport
  VTPM_S2IDLock_flg : Outport  Port=2
  Used : Outport  Port=3
  VTPM_LFS2_cnt : Outport  Port=4
  VTPM_RFS2_cnt : Outport  Port=5
  VTPM_LRS2_cnt : Outport  Port=6
  VTPM_RRS2_cnt : Outport  Port=7
  C : Outport  Port=8
  GS2 : Outport  Port=9
  VTPM_S2timeout_flg : Outport  Port=10
  wires:
  VPMM_PowerSta_enum/1 -> Chart/2(VPMM_PowerSta_enum)
  Constant18/1 -> Switch5/1
  [VINP_TPMSResButt_flg] -> Switch5/2
  Data Type Conversion10/1 -> Add/1
  Unit Delay1/1 -> Add/2
  Switch5/1 -> [VTPM_GS2_cnt], Unit Delay1/1  "VTPM_GS2_cnt"
  Add/1 -> Switch5/3
  [C] -> Detect Increase/1
  Enabled Subsystem3/1(S) -> VTPM_RRS2_cnt/1
  Enabled Subsystem2/1(S) -> VTPM_LRS2_cnt/1
  Enabled Subsystem1/1(S) -> VTPM_RFS2_cnt/1
  [C] -> C/1
  Enabled Subsystem5/1(S) -> VTPM_LFS2_cnt/1
  Chart/3(RRM) -> Enabled Subsystem3/2(LFM1)
  [Cal] -> Enabled Subsystem3/Enable
  [C] -> Enabled Subsystem3/1(C)
  [C] -> Enabled Subsystem2/1(C)
  [Cal] -> Enabled Subsystem2/Enable
  Chart/2(LRM) -> Enabled Subsystem2/2(LFM1)
  Chart/4(RFM) -> Enabled Subsystem1/2(LFM1)
  [Cal] -> Enabled Subsystem1/Enable
  [C] -> Enabled Subsystem1/1(C)
  [C] -> Enabled Subsystem5/1(C)
  VINP_IDin_raw32/1 -> [VINP_IDin_raw32]
  VINP_TPMSResButt_flg/1 -> [VINP_TPMSResButt_flg]
  [VINP_TPMSResButt_flg] -> Logical Operator/2
  VTPM_RFWP_raw16/1 -> Chart/7(RF_PC)
  VTPM_RRWP_raw16/1 -> Chart/6(RR_PC)
  VTPM_LFWP_raw16/1 -> Chart/5(LF_PC)
  VTPM_LRWP_raw16/1 -> Chart/4(LR_PC)
  [G] -> Chart/3(GS)
  [VINP_TPMSResButt_flg] -> Chart1/2(VINP_TPMSResButt_flg)
  [VTPM_S2IDLock_flg] -> VTPM_S2IDLock_flg/1
  [VINP_IDin_raw32] -> Chart1/1(VINP_IDin_raw32)
  VINP_DATAin_flg/1 -> Chart1/3(VINP_DATAin_flg)
  Chart1/4(IDout) -> IDOut/1
  Chart1/1(G) -> GS2/1, [G], Data Type Conversion10/1
  Chart1/3(VTPM_S2IDLock_flg) -> [VTPM_S2IDLock_flg]
  Chart1/2(Used) -> [Used]
  [Used] -> Used/1
  Logical Operator/1 -> Chart/1(VINP_TPMSResButt_flg)
  [Used] -> NOT/1
  NOT/1 -> Logical Operator/1
  Chart/5(C) -> [C]
  [Cal] -> Enabled Subsystem5/Enable
  Chart/1(LFM) -> Enabled Subsystem5/2(LFM1)
  Detect Increase/1 -> [Cal]
  Relational Operator/1 -> [VTPM_FlashIDlock_flg]
  Constant/1 -> Relational Operator/2
  VINP_S2ID_raw/1 -> Relational Operator/1, [VINP_S2ID_raw]
  VINP_VehSpeed_kph/1 -> Chart1/6(VINP_VehSpeed_kph)
  [VINP_S2ID_raw] -> Chart1/5(VINP_S2ID_raw)
  [VTPM_FlashIDlock_flg] -> Chart1/4(VTPM_FlashIDlock_flg)
  Chart1/5(VTPM_S2timeout_flg) -> VTPM_S2timeout_flg/1

== system tpm/TPM/TPMS/TPMS/Learn/AutoLocation/IDIdentify/Subsystem2 ==
  VINP_DATAin_flg : Inport
  VINP_TPMSResButt_flg : Inport  Port=2
  VINP_IDin_raw32 : Inport  Port=3
  VTPM_LFWP_raw16 : Inport  Port=4
  VTPM_RFWP_raw16 : Inport  Port=5
  VTPM_LRWP_raw16 : Inport  Port=6
  VTPM_RRWP_raw16 : Inport  Port=7
  VPMM_PowerSta_enum : Inport  Port=8
  VINP_VehSpeed_kph : Inport  Port=9
  VINP_S3ID_raw : Inport  Port=10
  Add : Sum
  Chart : Stateflow chart  TreatAsAtomicUnit=on
      settings: PortSchema="{\"entries\":[{\"content\":{\"sides\":[{\"content\":{\"connectorIds\":[\"In1\",\"In2\",\"In3\",\"In5\",\"In7\",\"In4\",\"In6\"]},\"type\":\"ConnectorPlacement.EquallySpacedRectSide\",\"uuid\":\"84bbdee3-6a13-4113-bc08-a0b87ba22909\"},{\"content\":{\"connectorIds\":[\"Out5\",\"Out1\",\"Out4\",\"Out2\",\"Out3\"],\"side\":\"RIGHT\"},\"type\":\"ConnectorPlacement.EquallySpacedRectSide\",\"uuid\":\"b8796851-ab69-429f-9540-9571864c98e0\"},{\"content\":{\"connectorIds\":[],\"side\":\"TOP\"},\"type\":\"ConnectorPlacement.EquallySpacedRectSide\",\"uuid\":\"52bdbec4-409e-4a9a-a4bb-373a9525aed8\"}]},\"type\":\"ConnectorPlacement.EquallySpacedConnector\",\"uuid\":\"6e0a7370-38f8-4d4e-a3e7-eb2ef4c24b0f\"}],\"packageUris\":[\"http://schema.mathworks.com/mf0/Connector/R2020b\"],\"version\":\"1.0\"}"
  Chart1 : Stateflow chart  TreatAsAtomicUnit=on
      settings: PortSchema="{\"entries\":[{\"content\":{\"sides\":[{\"content\":{\"connectorIds\":[\"In2\",\"In1\",\"In3\",\"In4\",\"In5\",\"In6\"]},\"type\":\"ConnectorPlacement.EquallySpacedRectSide\",\"uuid\":\"0106c0c7-b0dd-4985-8477-027279f2cfbe\"},{\"content\":{\"connectorIds\":[\"Out1\",\"Out2\",\"Out3\",\"Out4\",\"Out5\"],\"side\":\"RIGHT\"},\"type\":\"ConnectorPlacement.EquallySpacedRectSide\",\"uuid\":\"38b36b5e-8790-43f5-89a8-de723ff40088\"},{\"content\":{\"connectorIds\":[],\"side\":\"TOP\"},\"type\":\"ConnectorPlacement.EquallySpacedRectSide\",\"uuid\":\"aa12a430-979d-4bba-b5af-88414204d80d\"}]},\"type\":\"ConnectorPlacement.EquallySpacedConnector\",\"uuid\":\"9f6249c4-6459-404e-8830-3ea500254943\"}],\"packageUris\":[\"http://schema.mathworks.com/mf0/Connector/R2020b\"],\"version\":\"1.0\"}"
  Constant : Constant  Value=ZERO_INT
  Constant18 : Constant  Value=0
  Data Type Conversion10 : DataTypeConversion  OutDataTypeStr=uint32
  Detect Increase : simulink/Logic and Bit Operations/Detect Increase  vinit=0.0  OutDataTypeStr=boolean
  Enabled Subsystem1 : Subsystem  TreatAsAtomicUnit=on
  Enabled Subsystem2 : Subsystem  TreatAsAtomicUnit=on
  Enabled Subsystem3 : Subsystem  TreatAsAtomicUnit=on
  Enabled Subsystem5 : Subsystem  TreatAsAtomicUnit=on
  Logical Operator : Logic  Operator=OR  AllPortsSameDT=off  OutDataTypeStr=boolean
  NOT : Logic  Operator=NOT  IconShape=distinctive  AllPortsSameDT=off  OutDataTypeStr=boolean
  Relational Operator : RelationalOperator  Operator=~=  OutDataTypeStr=boolean  RndMeth=Simplest
  Switch5 : Switch  Criteria=u2 > Threshold
  Unit Delay1 : UnitDelay  SampleTime=-1  HasFrameUpgradeWarning=on
  IDOut : Outport
  VTPM_S3IDLock_flg : Outport  Port=2
  Used : Outport  Port=3
  VTPM_LFS3_cnt : Outport  Port=4
  VTPM_RFS3_cnt : Outport  Port=5
  VTPM_LRS3_cnt : Outport  Port=6
  VTPM_RRS3_cnt : Outport  Port=7
  C : Outport  Port=8
  GS3 : Outport  Port=9
  VTPM_S3timeout_flg : Outport  Port=10
  wires:
  Detect Increase/1 -> [Cal]
  Chart/1(LFM) -> Enabled Subsystem5/2(LFM1)
  [Cal] -> Enabled Subsystem5/Enable
  Chart/5(C) -> [C]
  NOT/1 -> Logical Operator/1
  [Used] -> NOT/1
  Logical Operator/1 -> Chart/1(VINP_TPMSResButt_flg)
  [Used] -> Used/1
  Chart1/2(Used) -> [Used]
  Chart1/3(VTPM_S3IDLock_flg) -> [VTPM_S3IDLock_flg]
  Chart1/1(G) -> [G], Data Type Conversion10/1, GS3/1
  Chart1/4(IDout) -> IDOut/1
  VINP_DATAin_flg/1 -> Chart1/3(VINP_DATAin_flg)
  [VINP_IDin_raw32] -> Chart1/1(VINP_IDin_raw32)
  [VTPM_S3IDLock_flg] -> VTPM_S3IDLock_flg/1
  [VINP_TPMSResButt_flg] -> Chart1/2(VINP_TPMSResButt_flg)
  [G] -> Chart/3(GS)
  VTPM_LRWP_raw16/1 -> Chart/4(LR_PC)
  VTPM_LFWP_raw16/1 -> Chart/5(LF_PC)
  VTPM_RRWP_raw16/1 -> Chart/6(RR_PC)
  VTPM_RFWP_raw16/1 -> Chart/7(RF_PC)
  [VINP_TPMSResButt_flg] -> Logical Operator/2
  VINP_TPMSResButt_flg/1 -> [VINP_TPMSResButt_flg]
  VINP_IDin_raw32/1 -> [VINP_IDin_raw32]
  [C] -> Enabled Subsystem5/1(C)
  [C] -> Enabled Subsystem1/1(C)
  [Cal] -> Enabled Subsystem1/Enable
  Chart/4(RFM) -> Enabled Subsystem1/2(LFM1)
  Chart/2(LRM) -> Enabled Subsystem2/2(LFM1)
  [Cal] -> Enabled Subsystem2/Enable
  [C] -> Enabled Subsystem2/1(C)
  [C] -> Enabled Subsystem3/1(C)
  [Cal] -> Enabled Subsystem3/Enable
  Chart/3(RRM) -> Enabled Subsystem3/2(LFM1)
  Enabled Subsystem5/1(S) -> VTPM_LFS3_cnt/1
  [C] -> C/1
  Enabled Subsystem1/1(S) -> VTPM_RFS3_cnt/1
  Enabled Subsystem2/1(S) -> VTPM_LRS3_cnt/1
  Enabled Subsystem3/1(S) -> VTPM_RRS3_cnt/1
  [C] -> Detect Increase/1
  Add/1 -> Switch5/3
  Switch5/1 -> Unit Delay1/1, [VTPM_GS3_cnt]  "VTPM_GS3_cnt"
  Unit Delay1/1 -> Add/2
  Data Type Conversion10/1 -> Add/1
  [VINP_TPMSResButt_flg] -> Switch5/2
  Constant18/1 -> Switch5/1
  VPMM_PowerSta_enum/1 -> Chart/2(VPMM_PowerSta_enum)
  Constant/1 -> Relational Operator/2
  VINP_S3ID_raw/1 -> Relational Operator/1, [VINP_S3ID_raw]
  Relational Operator/1 -> [VTPM_FlashIDlock_flg]
  VINP_VehSpeed_kph/1 -> Chart1/6(VINP_VehSpeed_kph)
  [VTPM_FlashIDlock_flg] -> Chart1/4(VTPM_FlashIDlock_flg)
  [VINP_S3ID_raw] -> Chart1/5(VINP_S3ID_raw)
  Chart1/5(VTPM_S3timeout_flg) -> VTPM_S3timeout_flg/1

== system tpm/TPM/TPMS/TPMS/Learn/AutoLocation/IDIdentify/Subsystem3 ==
  VINP_DATAin_flg : Inport
  VINP_TPMSResButt_flg : Inport  Port=2
  VINP_IDin_raw32 : Inport  Port=3
  VTPM_LFWP_raw16 : Inport  Port=4
  VTPM_RFWP_raw16 : Inport  Port=5
  VTPM_LRWP_raw16 : Inport  Port=6
  VTPM_RRWP_raw16 : Inport  Port=7
  VPMM_PowerSta_enum : Inport  Port=8
  VINP_VehSpeed_kph : Inport  Port=9
  VINP_S4ID_raw : Inport  Port=10
  Add : Sum
  Chart : Stateflow chart  TreatAsAtomicUnit=on
      settings: PortSchema="{\"entries\":[{\"content\":{\"sides\":[{\"content\":{\"connectorIds\":[\"In1\",\"In2\",\"In3\",\"In5\",\"In7\",\"In4\",\"In6\"]},\"type\":\"ConnectorPlacement.EquallySpacedRectSide\",\"uuid\":\"84bbdee3-6a13-4113-bc08-a0b87ba22909\"},{\"content\":{\"connectorIds\":[\"Out5\",\"Out1\",\"Out4\",\"Out2\",\"Out3\"],\"side\":\"RIGHT\"},\"type\":\"ConnectorPlacement.EquallySpacedRectSide\",\"uuid\":\"b8796851-ab69-429f-9540-9571864c98e0\"},{\"content\":{\"connectorIds\":[],\"side\":\"TOP\"},\"type\":\"ConnectorPlacement.EquallySpacedRectSide\",\"uuid\":\"52bdbec4-409e-4a9a-a4bb-373a9525aed8\"}]},\"type\":\"ConnectorPlacement.EquallySpacedConnector\",\"uuid\":\"6e0a7370-38f8-4d4e-a3e7-eb2ef4c24b0f\"}],\"packageUris\":[\"http://schema.mathworks.com/mf0/Connector/R2020b\"],\"version\":\"1.0\"}"
  Chart1 : Stateflow chart  TreatAsAtomicUnit=on
      settings: PortSchema="{\"entries\":[{\"content\":{\"sides\":[{\"content\":{\"connectorIds\":[\"In2\",\"In1\",\"In3\",\"In4\",\"In5\",\"In6\"]},\"type\":\"ConnectorPlacement.EquallySpacedRectSide\",\"uuid\":\"0106c0c7-b0dd-4985-8477-027279f2cfbe\"},{\"content\":{\"connectorIds\":[\"Out1\",\"Out2\",\"Out3\",\"Out4\",\"Out5\"],\"side\":\"RIGHT\"},\"type\":\"ConnectorPlacement.EquallySpacedRectSide\",\"uuid\":\"38b36b5e-8790-43f5-89a8-de723ff40088\"},{\"content\":{\"connectorIds\":[],\"side\":\"TOP\"},\"type\":\"ConnectorPlacement.EquallySpacedRectSide\",\"uuid\":\"aa12a430-979d-4bba-b5af-88414204d80d\"}]},\"type\":\"ConnectorPlacement.EquallySpacedConnector\",\"uuid\":\"9f6249c4-6459-404e-8830-3ea500254943\"}],\"packageUris\":[\"http://schema.mathworks.com/mf0/Connector/R2020b\"],\"version\":\"1.0\"}"
  Constant : Constant  Value=ZERO_INT
  Constant18 : Constant  Value=0
  Data Type Conversion10 : DataTypeConversion  OutDataTypeStr=uint32
  Detect Increase : simulink/Logic and Bit Operations/Detect Increase  vinit=0.0  OutDataTypeStr=boolean
  Enabled Subsystem1 : Subsystem  TreatAsAtomicUnit=on
  Enabled Subsystem2 : Subsystem  TreatAsAtomicUnit=on
  Enabled Subsystem3 : Subsystem  TreatAsAtomicUnit=on
  Enabled Subsystem5 : Subsystem  TreatAsAtomicUnit=on
  Logical Operator : Logic  Operator=OR  AllPortsSameDT=off  OutDataTypeStr=boolean
  NOT : Logic  Operator=NOT  IconShape=distinctive  AllPortsSameDT=off  OutDataTypeStr=boolean
  Relational Operator : RelationalOperator  Operator=~=  OutDataTypeStr=boolean  RndMeth=Simplest
  Switch5 : Switch  Criteria=u2 > Threshold
  Unit Delay1 : UnitDelay  SampleTime=-1  HasFrameUpgradeWarning=on
  IDOut : Outport
  VTPM_S4IDLock_flg : Outport  Port=2
  Used : Outport  Port=3
  VTPM_LFS4_cnt : Outport  Port=4
  VTPM_RFS4_cnt : Outport  Port=5
  VTPM_LRS4_cnt : Outport  Port=6
  VTPM_RRS4_cnt : Outport  Port=7
  C : Outport  Port=8
  GS4 : Outport  Port=9
  VTPM_S4timeout_flg : Outport  Port=10
  wires:
  VPMM_PowerSta_enum/1 -> Chart/2(VPMM_PowerSta_enum)
  Constant18/1 -> Switch5/1
  [VINP_TPMSResButt_flg] -> Switch5/2
  Data Type Conversion10/1 -> Add/1
  Unit Delay1/1 -> Add/2
  Switch5/1 -> [VTPM_GS4_cnt], Unit Delay1/1  "VTPM_GS4_cnt"
  Add/1 -> Switch5/3
  [C] -> Detect Increase/1
  Enabled Subsystem3/1(S) -> VTPM_RRS4_cnt/1
  Enabled Subsystem2/1(S) -> VTPM_LRS4_cnt/1
  Enabled Subsystem1/1(S) -> VTPM_RFS4_cnt/1
  [C] -> C/1
  Enabled Subsystem5/1(S) -> VTPM_LFS4_cnt/1
  Chart/3(RRM) -> Enabled Subsystem3/2(LFM1)
  [Cal] -> Enabled Subsystem3/Enable
  [C] -> Enabled Subsystem3/1(C)
  [C] -> Enabled Subsystem2/1(C)
  [Cal] -> Enabled Subsystem2/Enable
  Chart/2(LRM) -> Enabled Subsystem2/2(LFM1)
  Chart/4(RFM) -> Enabled Subsystem1/2(LFM1)
  [Cal] -> Enabled Subsystem1/Enable
  [C] -> Enabled Subsystem1/1(C)
  [C] -> Enabled Subsystem5/1(C)
  VINP_IDin_raw32/1 -> [VINP_IDin_raw32]
  VINP_TPMSResButt_flg/1 -> [VINP_TPMSResButt_flg]
  [VINP_TPMSResButt_flg] -> Logical Operator/2
  VTPM_RFWP_raw16/1 -> Chart/7(RF_PC)
  VTPM_RRWP_raw16/1 -> Chart/6(RR_PC)
  VTPM_LFWP_raw16/1 -> Chart/5(LF_PC)
  VTPM_LRWP_raw16/1 -> Chart/4(LR_PC)
  [G] -> Chart/3(GS)
  [VINP_TPMSResButt_flg] -> Chart1/2(VINP_TPMSResButt_flg)
  [VTPM_S4IDLock_flg] -> VTPM_S4IDLock_flg/1
  [VINP_IDin_raw32] -> Chart1/1(VINP_IDin_raw32)
  VINP_DATAin_flg/1 -> Chart1/3(VINP_DATAin_flg)
  Chart1/4(IDout) -> IDOut/1
  Chart1/1(G) -> GS4/1, [G], Data Type Conversion10/1
  Chart1/3(VTPM_S4IDLock_flg) -> [VTPM_S4IDLock_flg]
  Chart1/2(Used) -> [Used]
  [Used] -> Used/1
  Logical Operator/1 -> Chart/1(VINP_TPMSResButt_flg)
  [Used] -> NOT/1
  NOT/1 -> Logical Operator/1
  Chart/5(C) -> [C]
  [Cal] -> Enabled Subsystem5/Enable
  Chart/1(LFM) -> Enabled Subsystem5/2(LFM1)
  Detect Increase/1 -> [Cal]
  VINP_S4ID_raw/1 -> Relational Operator/1, [VINP_S4ID_raw]
  Constant/1 -> Relational Operator/2
  Relational Operator/1 -> [VTPM_FlashIDlock_flg]
  [VTPM_FlashIDlock_flg] -> Chart1/4(VTPM_FlashIDlock_flg)
  [VINP_S4ID_raw] -> Chart1/5(VINP_S4ID_raw)
  VINP_VehSpeed_kph/1 -> Chart1/6(VINP_VehSpeed_kph)
  Chart1/5(VTPM_S4timeout_flg) -> VTPM_S4timeout_flg/1

== system tpm/TPM/TPMS/TPMS/Learn/AutoLocation/IDIdentify/Subsystem7 ==
  VINP_DATAin_flg : Inport
  VINP_TPMSResButt_flg : Inport  Port=2
  VINP_IDin_raw32 : Inport  Port=3
  VTPM_LFWP_raw16 : Inport  Port=4
  VTPM_RFWP_raw16 : Inport  Port=5
  VTPM_LRWP_raw16 : Inport  Port=6
  VTPM_RRWP_raw16 : Inport  Port=7
  VPMM_PowerSta_enum : Inport  Port=8
  VINP_VehSpeed_kph : Inport  Port=9
  VINP_S1ID_raw : Inport  Port=10
  Add : Sum
  Chart : Stateflow chart  TreatAsAtomicUnit=on
      settings: PortSchema="{\"entries\":[{\"content\":{\"sides\":[{\"content\":{\"connectorIds\":[\"In1\",\"In2\",\"In3\",\"In5\",\"In7\",\"In4\",\"In6\"]},\"type\":\"ConnectorPlacement.EquallySpacedRectSide\",\"uuid\":\"84bbdee3-6a13-4113-bc08-a0b87ba22909\"},{\"content\":{\"connectorIds\":[\"Out5\",\"Out1\",\"Out4\",\"Out2\",\"Out3\"],\"side\":\"RIGHT\"},\"type\":\"ConnectorPlacement.EquallySpacedRectSide\",\"uuid\":\"b8796851-ab69-429f-9540-9571864c98e0\"},{\"content\":{\"connectorIds\":[],\"side\":\"TOP\"},\"type\":\"ConnectorPlacement.EquallySpacedRectSide\",\"uuid\":\"52bdbec4-409e-4a9a-a4bb-373a9525aed8\"}]},\"type\":\"ConnectorPlacement.EquallySpacedConnector\",\"uuid\":\"6e0a7370-38f8-4d4e-a3e7-eb2ef4c24b0f\"}],\"packageUris\":[\"http://schema.mathworks.com/mf0/Connector/R2020b\"],\"version\":\"1.0\"}"
  Chart1 : Stateflow chart  TreatAsAtomicUnit=on
      settings: PortSchema="{\"entries\":[{\"content\":{\"sides\":[{\"content\":{\"connectorIds\":[\"In2\",\"In1\",\"In3\",\"In4\",\"In5\",\"In6\"]},\"type\":\"ConnectorPlacement.EquallySpacedRectSide\",\"uuid\":\"0106c0c7-b0dd-4985-8477-027279f2cfbe\"},{\"content\":{\"connectorIds\":[\"Out1\",\"Out2\",\"Out3\",\"Out4\",\"Out5\"],\"side\":\"RIGHT\"},\"type\":\"ConnectorPlacement.EquallySpacedRectSide\",\"uuid\":\"38b36b5e-8790-43f5-89a8-de723ff40088\"},{\"content\":{\"connectorIds\":[],\"side\":\"TOP\"},\"type\":\"ConnectorPlacement.EquallySpacedRectSide\",\"uuid\":\"aa12a430-979d-4bba-b5af-88414204d80d\"}]},\"type\":\"ConnectorPlacement.EquallySpacedConnector\",\"uuid\":\"9f6249c4-6459-404e-8830-3ea500254943\"}],\"packageUris\":[\"http://schema.mathworks.com/mf0/Connector/R2020b\"],\"version\":\"1.0\"}"
  Constant : Constant  Value=ZERO_INT
  Constant18 : Constant  Value=0
  Data Type Conversion10 : DataTypeConversion  OutDataTypeStr=uint32
  Detect Increase : simulink/Logic and Bit Operations/Detect Increase  vinit=0.0  OutDataTypeStr=boolean
  Enabled Subsystem1 : Subsystem  TreatAsAtomicUnit=on
  Enabled Subsystem2 : Subsystem  TreatAsAtomicUnit=on
  Enabled Subsystem3 : Subsystem  TreatAsAtomicUnit=on
  Enabled Subsystem5 : Subsystem  TreatAsAtomicUnit=on
  Logical Operator : Logic  Operator=OR  AllPortsSameDT=off  OutDataTypeStr=boolean
  NOT : Logic  Operator=NOT  IconShape=distinctive  AllPortsSameDT=off  OutDataTypeStr=boolean
  Relational Operator : RelationalOperator  Operator=~=  OutDataTypeStr=boolean  RndMeth=Simplest
  Switch5 : Switch  Criteria=u2 > Threshold
  Unit Delay1 : UnitDelay  SampleTime=-1  HasFrameUpgradeWarning=on
  IDOut : Outport
  VTPM_S1IDLock_flg : Outport  Port=2
  Used : Outport  Port=3
  VTPM_LFS1_cnt : Outport  Port=4
  VTPM_RFS1_cnt : Outport  Port=5
  VTPM_LRS1_cnt : Outport  Port=6
  VTPM_RRS1_cnt : Outport  Port=7
  C : Outport  Port=8
  GS1 : Outport  Port=9
  VTPM_S1timeout_flg : Outport  Port=10
  wires:
  Detect Increase/1 -> [Cal]
  Chart/1(LFM) -> Enabled Subsystem5/2(LFM1)
  [Cal] -> Enabled Subsystem5/Enable
  Chart/5(C) -> [C]
  NOT/1 -> Logical Operator/1
  [Used] -> NOT/1
  Logical Operator/1 -> Chart/1(VINP_TPMSResButt_flg)
  [Used] -> Used/1
  Chart1/2(Used) -> [Used]
  Chart1/3(VTPM_S1IDLock_flg) -> [VTPM_S1IDLock_flg]
  Chart1/1(G) -> Data Type Conversion10/1, GS1/1, [G]
  Chart1/4(IDout) -> IDOut/1
  VINP_DATAin_flg/1 -> Chart1/3(VINP_DATAin_flg)
  [VINP_IDin_raw32] -> Chart1/1(VINP_IDin_raw32)
  [VTPM_S1IDLock_flg] -> VTPM_S1IDLock_flg/1
  [VINP_TPMSResButt_flg] -> Chart1/2(VINP_TPMSResButt_flg)
  [G] -> Chart/3(GS)
  VTPM_LRWP_raw16/1 -> Chart/4(LR_PC)
  VTPM_LFWP_raw16/1 -> Chart/5(LF_PC)
  VTPM_RRWP_raw16/1 -> Chart/6(RR_PC)
  VTPM_RFWP_raw16/1 -> Chart/7(RF_PC)
  [VINP_TPMSResButt_flg] -> Logical Operator/2
  VINP_TPMSResButt_flg/1 -> [VINP_TPMSResButt_flg]
  VINP_IDin_raw32/1 -> [VINP_IDin_raw32]
  [C] -> Enabled Subsystem5/1(C)
  [C] -> Enabled Subsystem1/1(C)
  [Cal] -> Enabled Subsystem1/Enable
  Chart/4(RFM) -> Enabled Subsystem1/2(LFM1)
  Chart/2(LRM) -> Enabled Subsystem2/2(LFM1)
  [Cal] -> Enabled Subsystem2/Enable
  [C] -> Enabled Subsystem2/1(C)
  [C] -> Enabled Subsystem3/1(C)
  [Cal] -> Enabled Subsystem3/Enable
  Chart/3(RRM) -> Enabled Subsystem3/2(LFM1)
  Enabled Subsystem5/1(S) -> VTPM_LFS1_cnt/1
  [C] -> C/1
  Enabled Subsystem1/1(S) -> VTPM_RFS1_cnt/1
  Enabled Subsystem2/1(S) -> VTPM_LRS1_cnt/1
  Enabled Subsystem3/1(S) -> VTPM_RRS1_cnt/1
  [C] -> Detect Increase/1
  Add/1 -> Switch5/3
  Switch5/1 -> Unit Delay1/1, [VTPM_GS1_cnt]  "VTPM_GS1_cnt"
  Unit Delay1/1 -> Add/2
  Data Type Conversion10/1 -> Add/1
  [VINP_TPMSResButt_flg] -> Switch5/2
  Constant18/1 -> Switch5/1
  VPMM_PowerSta_enum/1 -> Chart/2(VPMM_PowerSta_enum)
  VINP_VehSpeed_kph/1 -> Chart1/6(VINP_VehSpeed_kph)
  VINP_S1ID_raw/1 -> [VINP_S1ID_raw], Relational Operator/1
  Relational Operator/1 -> [VTPM_FlashIDlock_flg]
  Constant/1 -> Relational Operator/2
  [VTPM_FlashIDlock_flg] -> Chart1/4(VTPM_FlashIDlock_flg)
  [VINP_S1ID_raw] -> Chart1/5(VINP_S1ID_raw)
  Chart1/5(VTPM_S1timeout_flg) -> VTPM_S1timeout_flg/1
